simulink subsystem "EoM_Euler6DoF"  (R2024b)
settings: Solver=VariableStepAuto  StartTime=0.0  StopTime=10.0  RelTol=1e-3
undefined symbols (not defined in the file or in its folder): com_error, inertia_error, mass_error, vehicle
settings Model: Creator=thatf  LastModifiedBy=thatf

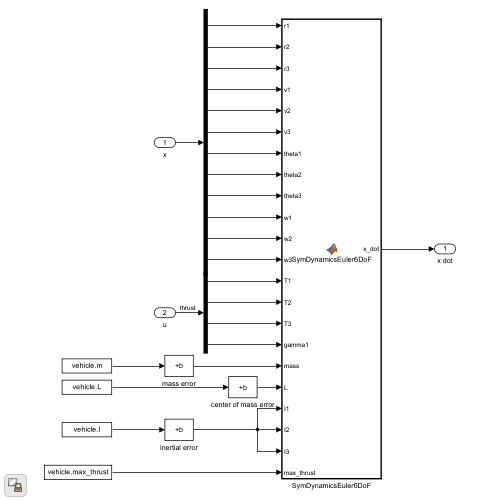
[thumbnail: Simulink's stored preview of the top-level diagram]
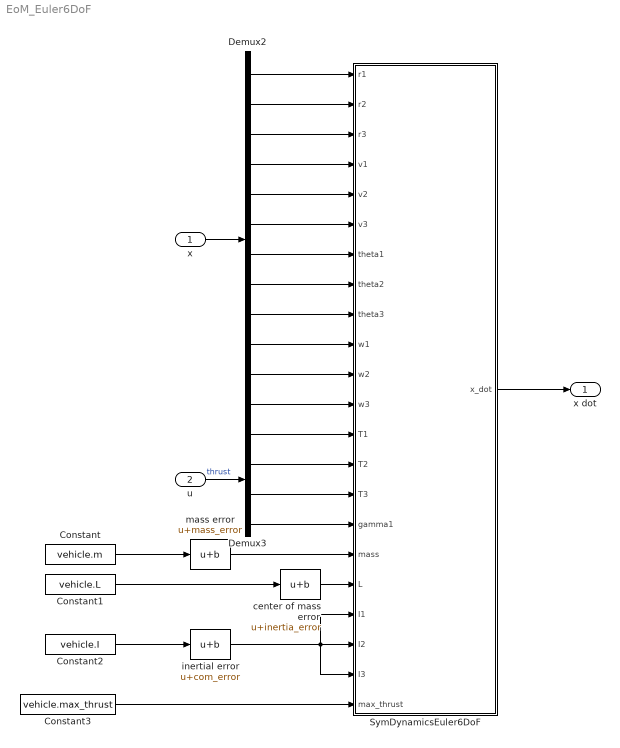
== system EoM_Euler6DoF ==
  x : Inport
  u : Inport  Port=2
  Constant : Constant  Value=vehicle.m
  Constant1 : Constant  Value=vehicle.L
  Constant2 : Constant  Value=vehicle.I
  Constant3 : Constant  Value=vehicle.max_thrust
  Demux2 : Demux  Outputs=dof.nx
  Demux3 : Demux  Outputs=dof.nu
  SymDynamicsEuler6DoF : MATLAB Function  TreatAsAtomicUnit=on
  center of mass error : Bias  Bias=inertia_error  SaturateOnIntegerOverflow=off
  inertial error : Bias  Bias=com_error  SaturateOnIntegerOverflow=off
  mass error : Bias  Bias=mass_error  SaturateOnIntegerOverflow=off
  x dot : Outport
  wires:
  x/1 -> Demux2/1
  Constant1/1 -> center of mass error/1
  Constant2/1 -> inertial error/1
  SymDynamicsEuler6DoF/1(x_dot) -> x dot/1
  u/1 -> Demux3/1  "thrust"
  mass error/1 -> SymDynamicsEuler6DoF/17(mass)
  Constant/1 -> mass error/1
  center of mass error/1 -> SymDynamicsEuler6DoF/18(L)
  Demux3/1 -> SymDynamicsEuler6DoF/13(T1)
  Demux2/11 -> SymDynamicsEuler6DoF/11(w2)
  Demux2/10 -> SymDynamicsEuler6DoF/10(w1)
  Demux2/9 -> SymDynamicsEuler6DoF/9(theta3)
  Demux2/8 -> SymDynamicsEuler6DoF/8(theta2)
  Demux2/1 -> SymDynamicsEuler6DoF/1(r1)
  Demux2/2 -> SymDynamicsEuler6DoF/2(r2)
  Demux2/3 -> SymDynamicsEuler6DoF/3(r3)
  Demux2/4 -> SymDynamicsEuler6DoF/4(v1)
  Demux2/5 -> SymDynamicsEuler6DoF/5(v2)
  Demux2/6 -> SymDynamicsEuler6DoF/6(v3)
  Demux2/7 -> SymDynamicsEuler6DoF/7(theta1)
  Demux3/2 -> SymDynamicsEuler6DoF/14(T2)
  Demux3/3 -> SymDynamicsEuler6DoF/15(T3)
  Constant3/1 -> SymDynamicsEuler6DoF/22(max_thrust)
  Demux2/12 -> SymDynamicsEuler6DoF/12(w3)
  Demux3/4 -> SymDynamicsEuler6DoF/16(gamma1)
  inertial error/1 -> SymDynamicsEuler6DoF/20(I2), SymDynamicsEuler6DoF/19(I1), SymDynamicsEuler6DoF/21(I3)

== matlab function EoM_Euler6DoF/SymDynamicsEuler6DoF ==
  data: r1 input; x_dot output; r2 input; r3 input; v1 input; v2 input; v3 input; theta1 input; theta2 input; theta3 input; w1 input; w2 input; w3 input; T1 input; T2 input; T3 input; gamma1 input; mass input; L input; I1 input; I2 input; I3 input; max_thrust input
function x_dot = SymDynamicsEuler6DoF(r1,r2,r3,v1,v2,v3,theta1,theta2,theta3,w1,w2,w3,T1,T2,T3,gamma1,mass,L,I1,I2,I3,max_thrust)
%#codegen

%    This function was generated by the Symbolic Math Toolbox version 24.2.
%    29-Dec-2024 21:01:45

% r1 = complex(r1);  % if required to enforce complex operations
% r2 = complex(r2);  % if required to enforce complex operations
% r3 = complex(r3);  % if required to enforce complex operations
% v1 = complex(v1);  % if required to enforce complex operations
% v2 = complex(v2);  % if required to enforce complex operations
% v3 = complex(v3);  % if required to enforce complex operations
% theta1 = complex(theta1);  % if required to enforce complex operations
% theta2 = complex(theta2);  % if required to enforce complex operations
% theta3 = complex(theta3);  % if required to enforce complex operations
% w1 = complex(w1);  % if required to enforce complex operations
% w2 = complex(w2);  % if required to enforce complex operations
% w3 = complex(w3);  % if required to enforce complex operations
% T1 = complex(T1);  % if required to enforce complex operations
% T2 = complex(T2);  % if required to enforce complex operations
% T3 = complex(T3);  % if required to enforce complex operations
% gamma1 = complex(gamma1);  % if required to enforce complex operations
% mass = complex(mass);  % if required to enforce complex operations
% L = complex(L);  % if required to enforce complex operations
% I1 = complex(I1);  % if required to enforce complex operations
% I2 = complex(I2);  % if required to enforce complex operations
% I3 = complex(I3);  % if required to enforce complex operations
% max_thrust = complex(max_thrust);  % if required to enforce complex operations
t2 = cos(gamma1);
t3 = cos(theta1);
t4 = cos(theta2);
t5 = cos(theta3);
t6 = sin(theta1);
t7 = sin(theta2);
t8 = sin(theta3);
t9 = -I3;
t10 = 1.0./mass;
t11 = 1.0./t7;
mt1 = [v1;v2;v3;t2.*t10.*(T1.*max_thrust.*t4+T3.*max_thrust.*t5.*t7+T2.*max_thrust.*t7.*t8);t2.*t10.*(T2.*max_thrust.*(t3.*t5-t4.*t6.*t8)-T3.*max_thrust.*(t3.*t8+t4.*t5.*t6)+T1.*max_thrust.*t6.*t7);-t2.*t10.*(-T2.*max_thrust.*(t5.*t6+t3.*t4.*t8)+T3.*max_thrust.*(t6.*t8-t3.*t4.*t5)+T1.*max_thrust.*t3.*t7)-9.81e+2./1.0e+2;t5.*t11.*w3+t8.*t11.*w2;t5.*w2-t8.*w3;w1-t4.*t5.*t11.*w3-t4.*t8.*t11.*w2;(sin(gamma1).*sqrt(abs(T1.*max_thrust).^2+abs(T2.*max_thrust).^2+abs(T3.*max_thrust).^2)+w2.*w3.*(I2+t9))./I1;-(w1.*w3.*(I1+t9)-L.*T3.*max_thrust.*t2)./I2];
mt2 = [(w1.*w2.*(I1-I2)-L.*T2.*max_thrust.*t2)./I3];
x_dot = [mt1;mt2];
end
